simulink model "heating_mechanism_radiator"  (R2016b)
settings: Solver=VariableStepAuto  StartTime=0.0  StopTime=10.0  RelTol=1e-3
libraries: simulink x1, cstblocks x1
settings Model: Creator=gylaszlo  LastModifiedBy=gylaszlo

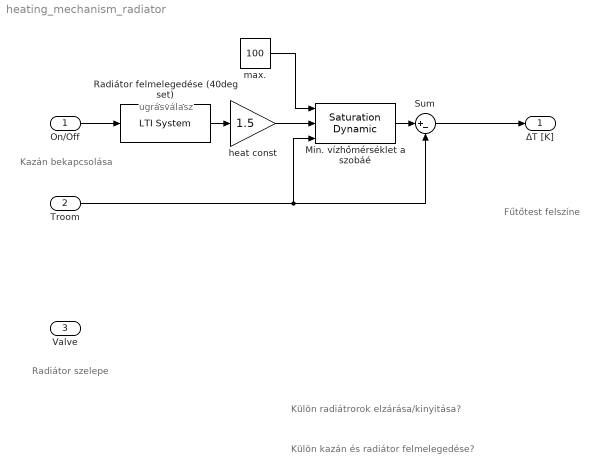
== system heating_mechanism_radiator ==
  note: Külön kazán és radiátor felmelegedése?
  note: Külön radiátrorok elzárása/kinyitása?
  note: ugrásválasz
  note: Radiátor szelepe
  note: Kazán bekapcsolása
  note: Fűtőtest felszíne
  On/Off : Inport
  Troom : Inport  Port=2
  Valve : Inport  Port=3
  Min. vízhőmérséklet a szobáé : simulink/Discontinuities/Saturation Dynamic  OutMin=[]  OutMax=[]  OutDataTypeStr=Inherit: Same as second input  OutDataType=fixdt(1, 16)  OutScaling=2^-10  DoSatur=off
  Radiátor felmelegedése (40deg set) : cstblocks/LTI System  sys=radiator_felulet  IC=[]
  Sum : Sum  Inputs=|+-
  heat const : Gain  Gain=1.5
  max. : Constant  Value=100
  ΔT [K] : Outport
  wires:
  On/Off/1 -> Radiátor felmelegedése (40deg set)/1
  Troom/1 -> Sum/2, Min. vízhőmérséklet a szobáé/3
  Radiátor felmelegedése (40deg set)/1 -> heat const/1
  max./1 -> Min. vízhőmérséklet a szobáé/1
  Min. vízhőmérséklet a szobáé/1 -> Sum/1
  heat const/1 -> Min. vízhőmérséklet a szobáé/2
  Sum/1 -> ΔT [K]/1
